simulink model "BLDCmotorControl_FOC_R2017b_fixdt_Ffwd"  (R2025a)
settings: Solver=FixedStepDiscrete  StartTime=0  StopTime=0.5  FixedStep=Ts  MaxStep=1e-6  RelTol=1e-6  AbsTol=1e-6  EnableMultiTasking=on
PreLoadFcn:
  | addpath(genpath('01_Libraries'));
  | addpath(genpath('02_Figures'));
InitFcn:
  | init_model;
undefined symbols (not defined in the file): a_elecAngle, b_DCLinkCurrAvail, b_diagEna, b_FfwdEna, b_fieldWeakEna, b_selPhaABCurrMeas, cf_currFilt, cf_speedCoef, cf_speedFilt, CTRL_COM, DiscIntNeverNeededParam, dV_openRate, DWORK0, DWORK1, DWORK2, DWORK3, dz_cntTrnsDetHi, dz_cntTrnsDetLo, i_errThres, i_max, i_thresOutlier, id_fieldWeak_M1, id_Kb, id_Ki, id_Kp, iq_Kb, iq_Ki, iq_KiLimProt, iq_Kp, iq_KpLimProt, iq_max_M1, Ld, Lq, mot_lambda, mot_Ld, mot_Lq, n_commAcvLo, n_commDeacvHi, n_Kb, n_Ki, n_Kp, n_KpLimProt, n_max, n_stdStillDet, OPEN_MODE, r_cos_M1, r_sin_M1, r_whl, Rs, SPD_MODE, t_errDequal, t_errQual, TRQ_MODE, Ts, Ts_ctrl, V_max, V_min, Vd_max, vec_hallToPos, VLT_MODE ... (+5)
libraries: BLDC_controller_Lib x12, simulink x11, spsPermanentMagnetSynchronousMachineLib x4, spsVoltageMeasurementLib x4, spsControlledVoltageSourceLib x2, spsUniversalBridgeLib x2, spspowerguiLib x2, eePwmGenerator x1, SignalEditorBlockLib x1
(part 4 of 4)

== stateflow chart BLDCmotorControl_FOC_R2017b_fixdt_Ffwd/BLDC_controller/BLDC_controller/F03_Control_Mode_Manager/F02_02_Control_Mode_Manager ==
  state OPEN
    entry:
    z_ctrlMod = OPEN_MODE;
  state ACTIVE
    state TORQUE_MODE
      entry:
      z_ctrlMod = TRQ_MODE;
    state SPEED_MODE
      entry:
      z_ctrlMod = SPD_MODE;
    state VOLTAGE_MODE
      entry:
      z_ctrlMod = VLT_MODE;
    (default) -> (junction 7)
    (junction 7) -> TORQUE_MODE [order 1] : [b_toTrqMod]
    (junction 7) -> (junction 8) [order 2]
    (junction 8) -> SPEED_MODE [order 1] : [b_toSpdMod]
    (junction 8) -> (junction 29) [order 2]
    (junction 29) -> VOLTAGE_MODE
  (default) -> OPEN
  OPEN -> ACTIVE : [b_toActive]
  ACTIVE -> OPEN : [b_toOpen]
  data: b_toOpen input boolean; b_toActive input boolean; b_toSpdMod input boolean; z_ctrlMod output uint8; OPEN_MODE constant uint8 =OPEN_MODE; TRQ_MODE constant uint8 =TRQ_MODE; SPD_MODE constant uint8 =SPD_MODE; VLT_MODE constant uint8 =VLT_MODE; b_toTrqMod input boolean
